simulink model "Example1"  (R2023b)
settings: Solver=VariableStepAuto  StartTime=0.0  StopTime=10.0  RelTol=1e-3
settings Model: Creator=The MathWorks, Inc.  LastModifiedBy=admin
settings SolverCC: MaxZcPerStep=1
settings DebuggingCC: UnconnectedInputMsg=warning  UnconnectedOutputMsg=warning  UnconnectedLineMsg=warning
settings ModelReferenceCC: EnableRefExpFcnMdlSchedulingChecks=on
settings RTWCC: DLArmComputeVersion=19.05

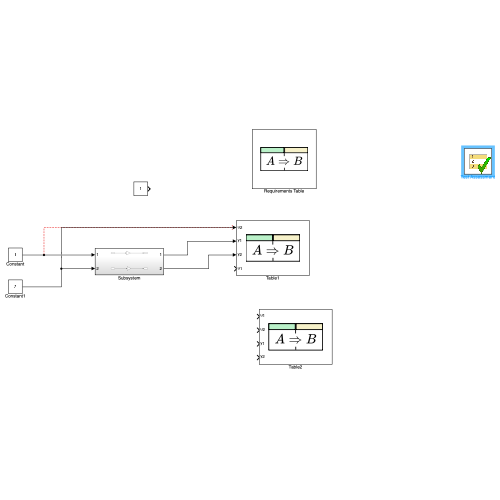
[thumbnail: Simulink's stored preview of the top-level diagram]
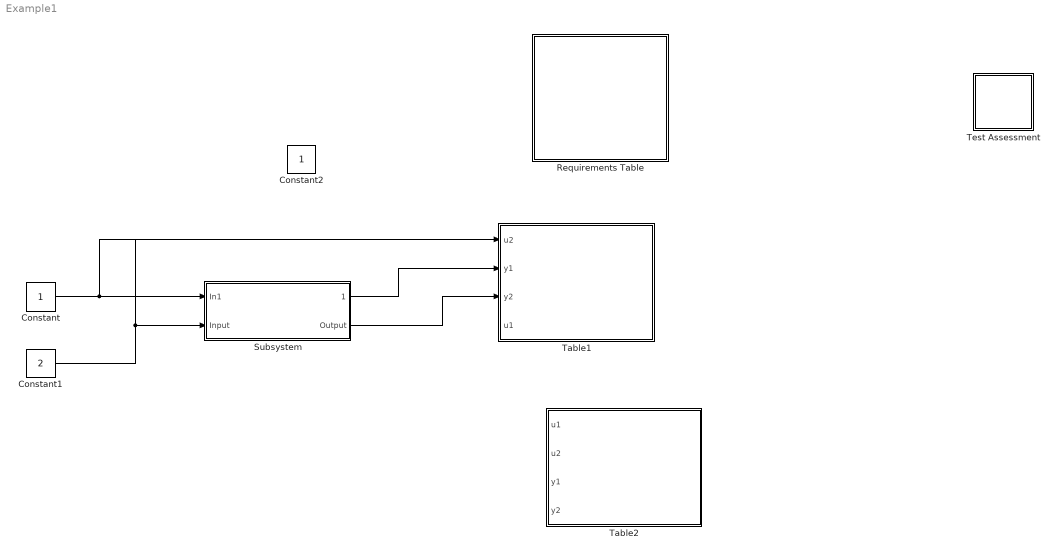
== system Example1 ==
  Constant : Constant
  Constant1 : Constant  Value=2
  Constant2 : Constant
  Requirements Table : Requirements Table  TreatAsAtomicUnit=on
  Subsystem : Subsystem
  Table1 : Requirements Table  TreatAsAtomicUnit=on
  Table2 : Requirements Table  TreatAsAtomicUnit=on
  Test Assessment : Test Sequence  TreatAsAtomicUnit=on
  wires:
  Subsystem/2(Output) -> Table1/3(y2)
  Constant/1 -> Subsystem/1(In1)
  Constant1/1 -> Subsystem/2(Input), Table1/1(u2)
  Subsystem/1(1) -> Table1/2(y1)

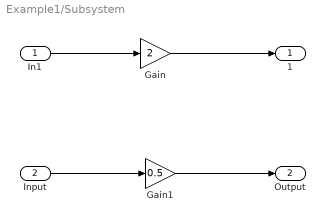
== system Example1/Subsystem ==
  In1 : Inport
  Input : Inport  Port=2
  Gain : Gain  Gain=2
  Gain1 : Gain  Gain=0.5
  1 : Outport
  Output : Outport  Port=2
  wires:
  Gain/1 -> 1/1
  In1/1 -> Gain/1
  Input/1 -> Gain1/1
  Gain1/1 -> Output/1

== stateflow chart Example1/Table2 ==
  (default) -> (junction 1073742791)
  (junction 1073742791) -> (junction 1073742792) : {
      | % SF_REQ_REV_07
      | }
  (junction 1073742792) -> (junction 1073742794) : {
      | % HEADER_ASSIGNMENTS
      |
      | }
  (junction 1073742794) -> (junction 1073742796) : {
      | % START_A_4
      | }
  (junction 1073742796) -> (junction 1073742798) : {
      | }
  (junction 1073742798) -> (junction 1073742800)
  (junction 1073742800) -> (junction 1073742802) : {
      | }
  (junction 1073742802) -> (junction 1073742804) : {
      | % END_A_4
      | }
  (junction 1073742804) -> (junction 1073742806) : {
      | % START_R_7
      | }
  (junction 1073742806) -> (junction 1073742808) : {
      | }
  (junction 1073742808) -> (junction 1073742810)
  (junction 1073742810) -> (junction 1073742812) [order 1] : [(u1==prev(u1)+1)]
  (junction 1073742810) -> (junction 1073742818) [order 2]
  (junction 1073742812) -> (junction 1073742814) : {
      | reqtable_postcondition((y1 == prev(y1)+2), 'R:1');
      |
      |
      | }
  (junction 1073742814) -> (junction 1073742816) : {
      | }
  (junction 1073742816) -> (junction 1073742818)
  (junction 1073742818) -> (junction 1073742820)
  (junction 1073742820) -> (junction 1073742822) : {
      | % END_R_7
      | }
  (junction 1073742822) -> (junction 1073742824) : {
      | % START_R_1
      | }
  (junction 1073742824) -> (junction 1073742826) : {
      | }
  (junction 1073742826) -> (junction 1073742828)
  (junction 1073742828) -> (junction 1073742830) [order 1] : [(u2 > 2)]
  (junction 1073742828) -> (junction 1073742836) [order 2]
  (junction 1073742830) -> (junction 1073742832) : {
      | reqtable_postcondition((y2 > 5), 'R:2');
      |
      |
      | }
  (junction 1073742832) -> (junction 1073742834) : {
      | }
  (junction 1073742834) -> (junction 1073742836)
  (junction 1073742836) -> (junction 1073742838)
  (junction 1073742838) -> (junction 1073742840) : {
      | % END_R_1
      | }
  data: u1 input double; u2 input double; y1 input double; y2 input double

== stateflow chart Example1/Requirements Table ==
  (default) -> (junction 1073741860)
  (junction 1073741860) -> (junction 1073741861) : {
      | % SF_REQ_REV_07
      | }
  (junction 1073741861) -> (junction 1073741863) : {
      | % HEADER_ASSIGNMENTS
      |
      | }
  (junction 1073741863) -> (junction 1073741865) : {
      | % START_A_4
      | }
  (junction 1073741865) -> (junction 1073741867) : {
      | }
  (junction 1073741867) -> (junction 1073741869)
  (junction 1073741869) -> (junction 1073741871) : {
      | }
  (junction 1073741871) -> (junction 1073741873) : {
      | % END_A_4
      | }
  (junction 1073741873) -> (junction 1073741898) : {
      | % START_R_1
      | }
  (junction 1073741898) -> (junction 1073741900) : {
      | }
  (junction 1073741900) -> (junction 1073741902) : {
      |
      |
      | }
  (junction 1073741902) -> (junction 1073741904) : {
      | }
  (junction 1073741904) -> (junction 1073741906) : {
      | % END_R_1
      | }

== stateflow chart Example1/Table1 ==
  (default) -> (junction 1073742791)
  (junction 1073742791) -> (junction 1073742792) : {
      | % SF_REQ_REV_07
      | }
  (junction 1073742792) -> (junction 1073742794) : {
      | % HEADER_ASSIGNMENTS
      |
      | }
  (junction 1073742794) -> (junction 1073742796) : {
      | % START_A_4
      | }
  (junction 1073742796) -> (junction 1073742798) : {
      | }
  (junction 1073742798) -> (junction 1073742800)
  (junction 1073742800) -> (junction 1073742802) : {
      | }
  (junction 1073742802) -> (junction 1073742804) : {
      | % END_A_4
      | }
  (junction 1073742804) -> (junction 1073742806) : {
      | % START_R_7
      | }
  (junction 1073742806) -> (junction 1073742808) : {
      | }
  (junction 1073742808) -> (junction 1073742810)
  (junction 1073742810) -> (junction 1073742812) [order 1] : [(u1==prev(u1)+1)]
  (junction 1073742810) -> (junction 1073742818) [order 2]
  (junction 1073742812) -> (junction 1073742814) : {
      | reqtable_postcondition((y1 == prev(y1)+2), 'R:1');
      |
      |
      | }
  (junction 1073742814) -> (junction 1073742816) : {
      | }
  (junction 1073742816) -> (junction 1073742818)
  (junction 1073742818) -> (junction 1073742820)
  (junction 1073742820) -> (junction 1073742822) : {
      | % END_R_7
      | }
  (junction 1073742822) -> (junction 1073742824) : {
      | % START_R_1
      | }
  (junction 1073742824) -> (junction 1073742826) : {
      | }
  (junction 1073742826) -> (junction 1073742828)
  (junction 1073742828) -> (junction 1073742830) [order 1] : [(u2 > 2)]
  (junction 1073742828) -> (junction 1073742836) [order 2]
  (junction 1073742830) -> (junction 1073742832) : {
      | reqtable_postcondition((y2 > 5), 'R:2');
      |
      |
      | }
  (junction 1073742832) -> (junction 1073742834) : {
      | }
  (junction 1073742834) -> (junction 1073742836)
  (junction 1073742836) -> (junction 1073742838)
  (junction 1073742838) -> (junction 1073742840) : {
      | % END_R_1
      | }
  data: u2 input double; y1 input double; y2 input double; u1 input double; data local

== stateflow chart Example1/Test Assessment ==
  state step_1
    state step_1_1
    state step_1_2
    (default) -> (junction 22)
    step_1 -> (junction 22)
    (junction 22) -> (junction 23) [order 1] : [HECATE_PARAM < 5
        | ]
    (junction 23) -> step_1_1 [order 1] : [~in(step_1.step_1_1)]
    (junction 23) -> (junction 26) [order 2]
    (junction 31) -> (junction 32)
    (junction 32) -> step_1_2 [order 1] : [~in(step_1.step_1_2)]
    (junction 32) -> (junction 35) [order 2]
    (junction 22) -> (junction 31) [order 2]
  (default) -> step_1
  data: HECATE_PARAM parameter
